simulink model "MMAE_beh_id_with_rel_LC_and_NGSIMTrajectories"  (R2018b)
settings: Solver=FixedStepAuto  StartTime=0.0  StopTime=90  FixedStep=Ts_bp  RelTol=1e-3
values from neighbouring files (symbols this model uses):
  ax = 0    [initialization.m]
  P_init = 1    [initialization.m]
  rel_x = 0    [initialization.m]
  Ts = 0.1    [KinematicBicycleModel.m]    (also in LeftLaneChangeSinusoidalMotionModel.m; LinearizedBicycleModel.m; SimplifiedKinematicBicycleModel.m; amm_rel_test.m)
  Ts_bp = 0.1    [initialization.m]    (also in laneChangeSinusoidalFcn.m = 0.01; laneChangeSinusoidalJacobianFcn.m = 0.01; leftLaneChangeParametricFcn.m = 0.01; leftLaneChangeParametricWithAccFcn.m = 0.01)
  vx = X(2)    [cv_model_fun.m]    (also in initialization.m = 10)
  vy = X(4)    [cv_model_fun.m]    (also in initialization.m = 0)
  x = X(1)    [KinematicBicycleModel.m]    (also in SimplifiedKinematicBicycleModel.m; behavior_model.m = 0:0.01:20; cca_model_fun.m; ctra_model_fun.m)
  y = X(2)    [KinematicBicycleModel.m]    (also in SimplifiedKinematicBicycleModel.m; behavior_model.m = [distances velocities]; cca_model_fun.m; ctra_model_fun.m)
undefined symbols (not defined in the file or in its folder): sigbuilder_block
libraries: simulink x8, dspswit3 x2, dspstat3 x2
settings Model: Creator=jasprit  LastModifiedBy=jasprit
settings SFSimCC: SimUseLocalCustomCode=off
settings RTWCC: RTWUseLocalCustomCode=off

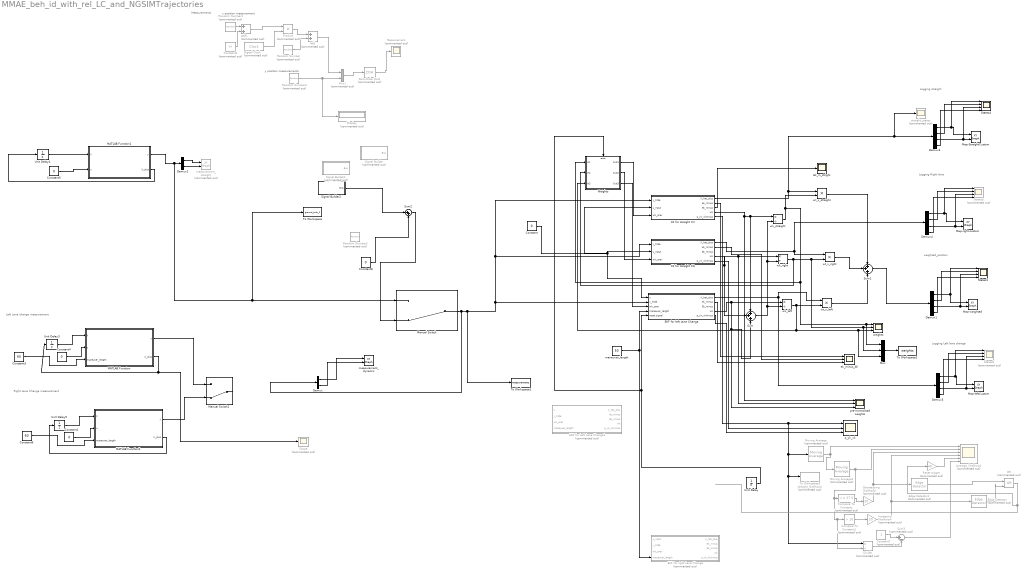
== system MMAE_beh_id_with_rel_LC_and_NGSIMTrajectories ==
  note: Left Lane change measurement
  note: Right Lane Change measurement
  note: Logging Left lane change
  note: Logging straight
  note: Logging Right lane
  note: y position measurements
  note: x position measurement
  note: Measurements
  note: weighted_position
  Add : Sum  Commented=on
  Add1 : Sum  Commented=on
  Average_likelihood : Scope  Commented=on  NumInputPorts=6
  Compare To Constant : simulink/Logic and Bit Operations/Compare To Constant  Commented=on  relop=<=  const=27.5  OutDataTypeStr=boolean
  Compare To Constant1 : simulink/Logic and Bit Operations/Compare To Constant  Commented=on  relop=>  const=10  OutDataTypeStr=boolean
  Constant : Constant  Value=0
  Constant1 : Constant  Value=0  SampleTime=-1
  Constant2 : Constant  Commented=on  Value=vx  SampleTime=Ts
  Constant3 : Constant  Value=60
  Constant4 : Constant  Value=0  SampleTime=-1
  Constant5 : Constant  Value=0  SampleTime=-1
  Constant6 : Constant  Value=60
  Constant7 : Constant  Commented=on
  Constant8 : Constant  Value=0
  Decreasomg likelihood : Gain  Commented=on  Gain=20
  Demux : Demux  Outputs=2
  Demux{1,3..5} (4 alike) : Demux
  Demux2 : Demux  Outputs=2
  Digital Clock : DigitalClock  Commented=on  SampleTime=Ts
  Display : Display  Commented=on
  Divide : Product  Commented=on  Inputs=*/
  EKF for Left Lane Change1 : Subsystem  Commented=on
  EKF for left Lane Change : Subsystem  TreatAsAtomicUnit=on
  EKF for right Lane Change : Subsystem  Commented=on
  Edge Detector : dspswit3/Edge Detector  Commented=on
      settings: SourceProductName=DSP System Toolbox  SourceProductBaseCode=DS
  Edge Detector1 : dspswit3/Edge Detector  Commented=on
      settings: SourceProductName=DSP System Toolbox  SourceProductBaseCode=DS
  Ek_m_stright : Scope
  Increasing likelihood : Gain  Commented=on  Gain=20
  KF for straight CA : Subsystem
  KF for straight CV : Subsystem
  MATLAB Function : MATLAB Function  TreatAsAtomicUnit=on
  MATLAB Function1 : MATLAB Function  TreatAsAtomicUnit=on
  MATLAB Function2 : MATLAB Function  TreatAsAtomicUnit=on
  Manual Switch : ManualSwitch  CurrentSetting=0
  Manual Switch1 : ManualSwitch  CurrentSetting=0
  Map-StraightCustom : simulink/Sinks/XY Graph  xmin=-1  xmax=200  ymin=-20  ymax=20  st=-1
  Map-leftCustom : simulink/Sinks/XY Graph  xmin=-1  xmax=300  ymin=-5  ymax=5  st=-1
  Map-right-custom : simulink/Sinks/XY Graph  xmin=-1  xmax=300  ymin=-5  ymax=5  st=-1
  Map-weighted : simulink/Sinks/XY Graph  xmin=-1  xmax=300  ymin=-5  ymax=5  st=-1
  "Measurement " : Scope  Commented=on
  Moving Average : dspstat3/Moving Average  Commented=on  Method=Sliding window  ForgettingFactorPort=off  SpecifyWindowLength=on  WindowLength=4  ForgettingFactor=0.9  SimulateUsing=Code generation
  Moving Average1 : dspstat3/Moving Average  Commented=on  Method=Sliding window  ForgettingFactorPort=off  SpecifyWindowLength=on  WindowLength=20  ForgettingFactor=0.9  SimulateUsing=Code generation
  Mux : Mux  Inputs=3
  Mux1 : Mux  Commented=on  Inputs=2
  OR : Logic  Commented=on  Operator=OR  IconShape=distinctive  AllPortsSameDT=off  OutDataTypeStr=boolean
  Product : Product  Commented=on
  Random Number : RandomNumber  Commented=on  Variance=0.0025  SampleTime=Ts
  Random Number1 : RandomNumber  Commented=on  Variance=0.0025  SampleTime=Ts
  Random Number2 : RandomNumber  Commented=on  Variance=0.0025  SampleTime=0.01
  Random Number3 : RandomNumber  Commented=on  Variance=0.0025  SampleTime=Ts
  Reset trigger : Gain  Commented=on  Gain=40
  Scope : Scope  Commented=on
  Signal Builder : Subsystem  Tag=STV Subsys  Commented=on  LoadFcn=sigbuilder_block('load');  StartFcn=sigbuilder_block('start');  StopFcn=sigbuilder_block('stop');  ClipboardFcn=sigbuilder_block('clipboard');  mask(Sigbuilder block){tuvar=[0:10]}
      mask help: Simulink:masks:SigbuilderBlock_MD
      mask init:
      | if ~strcmp(get_param(bdroot(gcbh),'SimulationStatus'),'stopped') tuvar = sigbuilder_block('maskInit'); end
      settings: CopyFcn=sigbuilder_block('copy');  DeleteFcn=sigbuilder_block('delete');  ModelCloseFcn=sigbuilder_block('modelClose');  PreSaveFcn=sigbuilder_block('preSave');  PauseFcn=sigbuilder_block('pause');  ContinueFcn=sigbuilder_block('continue');  NameChangeFcn=sigbuilder_block('namechange');  OpenFcn=sigbuilder_block('open',[414.75 96.75 558 422.25 ]);  CloseFcn=sigbuilder_block('close');
      mask Display: plot(0, 0, 100, 100,[2, 2, 32, 32, 2], [68, 8, 8, 68, 68],[32, 2], [38, 38], [32, 19, 2],[53, 60, 44], [32, 17, 17, 2],[16, 16, 31, 31]);txt = getActiveGroup(gcbh);text(2, 100, txt,'verticalAlignment', 'top');
  Signal Builder1 : Subsystem  Tag=STV Subsys  Commented=on  LoadFcn=sigbuilder_block('load');  StartFcn=sigbuilder_block('start');  StopFcn=sigbuilder_block('stop');  ClipboardFcn=sigbuilder_block('clipboard');  mask(Sigbuilder block){tuvar=[0:10]}
      mask help: Simulink:masks:SigbuilderBlock_MD
      mask init:
      | if ~strcmp(get_param(bdroot(gcbh),'SimulationStatus'),'stopped') tuvar = sigbuilder_block('maskInit'); end
      settings: CopyFcn=sigbuilder_block('copy');  DeleteFcn=sigbuilder_block('delete');  ModelCloseFcn=sigbuilder_block('modelClose');  PreSaveFcn=sigbuilder_block('preSave');  PauseFcn=sigbuilder_block('pause');  ContinueFcn=sigbuilder_block('continue');  NameChangeFcn=sigbuilder_block('namechange');  OpenFcn=sigbuilder_block('open',[492.75 131.25 580.5 283.5 ]);  CloseFcn=sigbuilder_block('close');
      mask Display: plot(0, 0, 100, 100,[2, 2, 32, 32, 2], [68, 8, 8, 68, 68],[32, 2], [38, 38], [32, 19, 2],[53, 60, 44], [32, 17, 17, 2],[16, 16, 31, 31]);txt = getActiveGroup(gcbh);text(2, 100, txt,'verticalAlignment', 'top');
  Signal Builder2 : Subsystem  Tag=STV Subsys  LoadFcn=sigbuilder_block('load');  StartFcn=sigbuilder_block('start');  StopFcn=sigbuilder_block('stop');  ClipboardFcn=sigbuilder_block('clipboard');  mask(Sigbuilder block){tuvar=[0:10]}
      mask help: Simulink:masks:SigbuilderBlock_MD
      mask init:
      | if ~strcmp(get_param(bdroot(gcbh),'SimulationStatus'),'stopped') tuvar = sigbuilder_block('maskInit'); end
      settings: CopyFcn=sigbuilder_block('copy');  DeleteFcn=sigbuilder_block('delete');  ModelCloseFcn=sigbuilder_block('modelClose');  PreSaveFcn=sigbuilder_block('preSave');  PauseFcn=sigbuilder_block('pause');  ContinueFcn=sigbuilder_block('continue');  NameChangeFcn=sigbuilder_block('namechange');  OpenFcn=sigbuilder_block('open',[437.6 178.5 550.15 399.75 ]);  CloseFcn=sigbuilder_block('close');
      mask Display: plot(0, 0, 100, 100,[2, 2, 32, 32, 2], [68, 8, 8, 68, 68],[32, 2], [38, 38], [32, 19, 2],[53, 60, 44], [32, 17, 17, 2],[16, 16, 31, 31]);txt = getActiveGroup(gcbh);text(2, 100, txt,'verticalAlignment', 'top');
  States1 : Scope  NumInputPorts=4
  States4 : Scope  NumInputPorts=4
  States5 : Scope  Commented=on  NumInputPorts=4
  States6 : Scope  Commented=on  NumInputPorts=4
  Sum : Sum  Inputs=+++
  Sum1 : Sum  Inputs=+++
  Sum2 : Sum  Inputs=|++
  Sum3 : Sum  Commented=on  Inputs=|+-
  To Workspace : ToWorkspace  VariableName=ground_truth_2  SaveFormat=Timeseries  SampleTime=-1
  To Workspace1 : ToWorkspace  VariableName=measurements  SaveFormat=Timeseries  SampleTime=-1
  To Workspace2 : ToWorkspace  VariableName=weights  SaveFormat=Timeseries  SampleTime=-1
  To Workspace3 : ToWorkspace  Commented=on  VariableName=straight_likelihood  SaveFormat=Timeseries  SampleTime=-1
  Unit Delay : UnitDelay  SampleTime=-1
  Unit Delay3 : UnitDelay  InitialCondition=[x vx y vy]  SampleTime=Ts_bp
  Unit Delay4 : UnitDelay  InitialCondition=[x vx y vy]  SampleTime=-1
  Unit Delay5 : UnitDelay  InitialCondition=[x vx y vy]  SampleTime=Ts_bp
  Weights : Subsystem
  Zero-Order Hold : ZeroOrderHold  Commented=on  SampleTime=Ts
  ek_minus_All : Scope  NumInputPorts=3
  maneuver_length : Constant  Value=50
  measurement_dynamic : simulink/Sinks/XY Graph  xmin=-1  xmax=700  ymin=-5  ymax=20  st=-1
  measurement_straight : simulink/Sinks/XY Graph  Commented=on  xmin=-1  xmax=200  ymin=-5  ymax=5  st=-1
  p_yk_xk : Scope  NumInputPorts=3
  pre-normalized weights : Scope  NumInputPorts=3
  straight_states : Scope  Commented=on
  weights : Scope  NumInputPorts=3
  wk_left : Product  Inputs=*/
  wk_right : Product  Inputs=*/
  wk_straight : Product  Inputs=*/
  wt_x_left : Product  Inputs=**
  wt_x_right : Product  Inputs=**
  wt_x_straight : Product  Inputs=**
  wires:
  Constant2/1 -> Add1/2
  Digital Clock/1 -> Product/2
  Product/1 -> Add/1
  Random Number/1 -> Add/2
  Add/1 -> Mux1/1
  Mux1/1 -> Zero-Order Hold/1
  Random Number3/1 -> Display/1, Mux1/2
  Zero-Order Hold/1 -> "Measurement "/1
  Demux3/1 -> States4/1, Map-StraightCustom/1
  Demux3/4 -> States4/4
  Demux3/2 -> States4/2
  Demux3/3 -> Map-StraightCustom/2, States4/3
  Constant/1 -> EKF for left Lane Change/1(u), KF for straight CA/2(u_input), KF for straight CV/2(u_input)
  Demux4/1 -> States5/1, Map-right-custom/1
  Demux4/2 -> States5/2
  Demux4/4 -> States5/4
  Demux4/3 -> Map-right-custom/2, States5/3
  Demux5/1 -> States6/1, Map-leftCustom/1
  Demux5/4 -> States6/4
  Demux5/3 -> Map-leftCustom/2, States6/3
  Demux5/2 -> States6/2
  EKF for left Lane Change/1(X_hat_plus) -> wt_x_left/1, Demux5/1
  KF for straight CA/1(X_hat_plus) -> Demux4/1, wt_x_right/1
  KF for straight CV/1(X_hat_plus) -> straight_states/1, Demux3/1, wt_x_straight/1
  EKF for left Lane Change/4(wk) -> wk_left/1, pre-normalized weights/3, Sum/3
  KF for straight CA/4(wk) -> pre-normalized weights/2, wk_right/1, Sum/2
  KF for straight CV/4(wk) -> pre-normalized weights/1, wk_straight/1, Sum/1
  Sum/1 -> wk_left/2, wk_straight/2, wk_right/2
  wk_straight/1 -> Weights/1(In1), Mux/1, weights/1, wt_x_straight/2
  wk_right/1 -> Weights/2(In2), Mux/2, weights/2, wt_x_right/2
  wk_left/1 -> Mux/3, weights/3, Weights/3(In3), wt_x_left/2
  wt_x_right/1 -> Sum1/2
  wt_x_straight/1 -> Sum1/1
  wt_x_left/1 -> Sum1/3
  Demux1/1 -> States1/1, Map-weighted/1
  Demux1/4 -> States1/4
  Demux1/2 -> States1/2
  Demux1/3 -> States1/3, Map-weighted/2
  Sum1/1 -> Demux1/1
  KF for straight CV/2(ek_minus) -> ek_minus_All/1
  KF for straight CA/2(ek_minus) -> ek_minus_All/2
  EKF for left Lane Change/2(ek_minus) -> ek_minus_All/3
  KF for straight CV/5(p_yk_xkminus) -> Moving Average/1, Divide/1, To Workspace3/1, p_yk_xk/1
  KF for straight CA/5(p_yk_xkminus) -> p_yk_xk/2
  EKF for left Lane Change/5(p_yk_xkminus) -> p_yk_xk/3
  KF for straight CV/3(Ek_minus) -> Ek_m_stright/1
  Manual Switch/1 -> To Workspace1/1, KF for straight CA/1(y_tilde), KF for straight CV/1(y_tilde), EKF for left Lane Change/2(y_tilde), Demux/1
  Unit Delay3/1 -> MATLAB Function/1(X)
  Constant4/1 -> MATLAB Function/2(u)
  Demux/1 -> measurement_dynamic/1
  Demux/2 -> measurement_dynamic/2
  MATLAB Function1/2(X_plus) -> Unit Delay4/1
  Constant5/1 -> MATLAB Function1/2(u)
  Unit Delay4/1 -> MATLAB Function1/1(X)
  MATLAB Function1/1(y) -> To Workspace/1, Manual Switch/1, Demux2/1
  Demux2/1 -> measurement_straight/1
  Demux2/2 -> measurement_straight/2
  MATLAB Function2/2(X_plus) -> Unit Delay5/1
  Unit Delay5/1 -> MATLAB Function2/1(X)
  Constant1/1 -> MATLAB Function2/2(u)
  MATLAB Function/1(y) -> Manual Switch1/1
  MATLAB Function2/1(y) -> Manual Switch1/2
  Random Number1/1 -> Add1/1
  Add1/1 -> Product/1
  maneuver_length/1 -> EKF for left Lane Change/4(maneuver_length), EKF for right Lane Change/4(maneuver_length)
  Constant3/1 -> MATLAB Function/3(maneuver_length)
  Constant6/1 -> MATLAB Function2/3(maneuver_length)
  MATLAB Function/2(X_plus) -> Scope/1, Unit Delay3/1
  Mux/1 -> To Workspace2/1
  Signal Builder2/1(Bus) -> Sum2/1
  Constant8/1 -> Sum2/2
  Sum2/1 -> Manual Switch/2
  Moving Average/1 -> Average_likelihood/1, Moving Average1/1
  Moving Average1/1 -> Divide/2, Compare To Constant1/1, Compare To Constant/1, Average_likelihood/2
  Decreasomg likelihood/1 -> Edge Detector1/1, Average_likelihood/3
  Unit Delay/1 -> Weights/Reset, EKF for left Lane Change/5(reset signal)
  Weights/1(Out1) -> KF for straight CV/3(wk_prev)
  Weights/2(Out2) -> KF for straight CA/3(wk_prev)
  Weights/3(Out3) -> EKF for left Lane Change/3(wk_prev)
  Compare To Constant/1 -> Decreasomg likelihood/1
  Compare To Constant1/1 -> Increasing likelihood/1
  Increasing likelihood/1 -> Edge Detector/1, Average_likelihood/4
  Edge Detector/1 -> OR/2
  Reset trigger/1 -> Average_likelihood/5
  Edge Detector1/1 -> OR/1
  OR/1 -> Reset trigger/1
  Constant7/1 -> Sum3/1
  Divide/1 -> Sum3/2
  Sum3/1 -> Average_likelihood/6

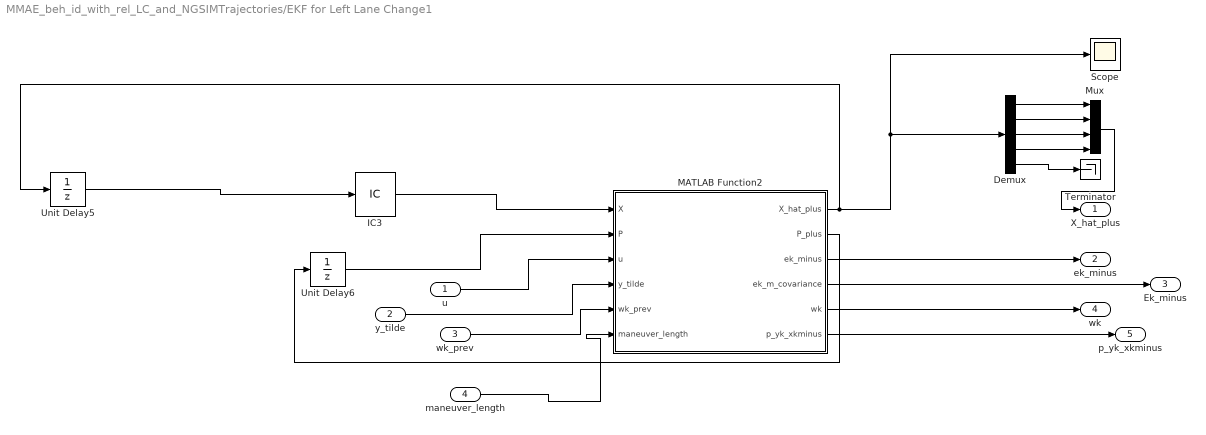
== system MMAE_beh_id_with_rel_LC_and_NGSIMTrajectories/EKF for Left Lane Change1 ==
  u : Inport
  y_tilde : Inport  Port=2
  wk_prev : Inport  Port=3
  maneuver_length : Inport  Port=4
  Demux : Demux  Outputs=5
  IC3 : InitialCondition  Value=[x vx y vy rel_x]
  MATLAB Function2 : MATLAB Function  TreatAsAtomicUnit=on
  Mux : Mux
  Scope : Scope
  Terminator : Terminator
  Unit Delay5 : UnitDelay  SampleTime=-1
  Unit Delay6 : UnitDelay  InitialCondition=diag([P_init, P_init, P_init, P_init, 200])  SampleTime=-1
  X_hat_plus : Outport
  ek_minus : Outport  Port=2
  Ek_minus : Outport  Port=3
  wk : Outport  Port=4
  p_yk_xkminus : Outport  Port=5
  wires:
  MATLAB Function2/2(P_plus) -> Unit Delay6/1
  u/1 -> MATLAB Function2/3(u)
  Unit Delay5/1 -> IC3/1
  y_tilde/1 -> MATLAB Function2/4(y_tilde)
  MATLAB Function2/1(X_hat_plus) -> Demux/1, Scope/1, Unit Delay5/1
  IC3/1 -> MATLAB Function2/1(X)
  Unit Delay6/1 -> MATLAB Function2/2(P)
  MATLAB Function2/3(ek_minus) -> ek_minus/1
  MATLAB Function2/4(ek_m_covariance) -> Ek_minus/1
  MATLAB Function2/5(wk) -> wk/1
  MATLAB Function2/6(p_yk_xkminus) -> p_yk_xkminus/1
  wk_prev/1 -> MATLAB Function2/5(wk_prev)
  maneuver_length/1 -> MATLAB Function2/6(maneuver_length)
  Demux/1 -> Mux/1
  Demux/2 -> Mux/2
  Demux/3 -> Mux/3
  Demux/4 -> Mux/4
  Demux/5 -> Terminator/1
  Mux/1 -> X_hat_plus/1

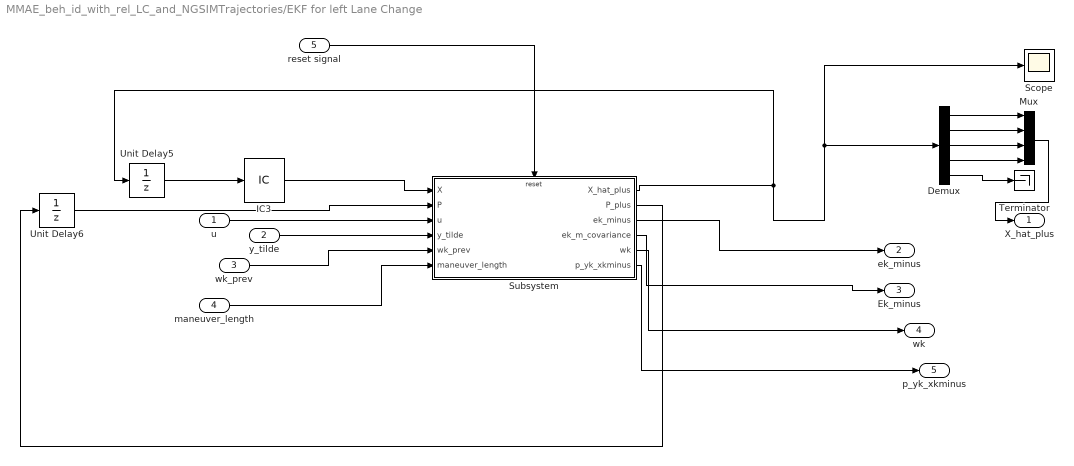
== system MMAE_beh_id_with_rel_LC_and_NGSIMTrajectories/EKF for left Lane Change ==
  u : Inport
  y_tilde : Inport  Port=2
  wk_prev : Inport  Port=3
  maneuver_length : Inport  Port=4
  reset signal : Inport  Port=5
  Demux : Demux  Outputs=5
  IC3 : InitialCondition  Value=[x vx y vy rel_x]
  Mux : Mux
  Scope : Scope
  Subsystem : Subsystem
  Terminator : Terminator
  Unit Delay5 : UnitDelay  InitialCondition=[x vx y vy rel_x]  SampleTime=-1
  Unit Delay6 : UnitDelay  InitialCondition=diag([P_init, P_init, P_init, P_init, 200])  SampleTime=-1
  X_hat_plus : Outport
  ek_minus : Outport  Port=2
  Ek_minus : Outport  Port=3
  wk : Outport  Port=4
  p_yk_xkminus : Outport  Port=5
  wires:
  Mux/1 -> X_hat_plus/1
  Demux/4 -> Mux/4
  Demux/5 -> Terminator/1
  Demux/3 -> Mux/3
  Demux/2 -> Mux/2
  Unit Delay5/1 -> IC3/1
  Demux/1 -> Mux/1
  Subsystem/1(X_hat_plus) -> Demux/1, Scope/1, Unit Delay5/1
  IC3/1 -> Subsystem/1(X)
  u/1 -> Subsystem/3(u)
  y_tilde/1 -> Subsystem/4(y_tilde)
  wk_prev/1 -> Subsystem/5(wk_prev)
  maneuver_length/1 -> Subsystem/6(maneuver_length)
  Subsystem/3(ek_minus) -> ek_minus/1
  Subsystem/4(ek_m_covariance) -> Ek_minus/1
  Subsystem/5(wk) -> wk/1
  Subsystem/6(p_yk_xkminus) -> p_yk_xkminus/1
  Unit Delay6/1 -> Subsystem/2(P)
  Subsystem/2(P_plus) -> Unit Delay6/1
  reset signal/1 -> Subsystem/Reset

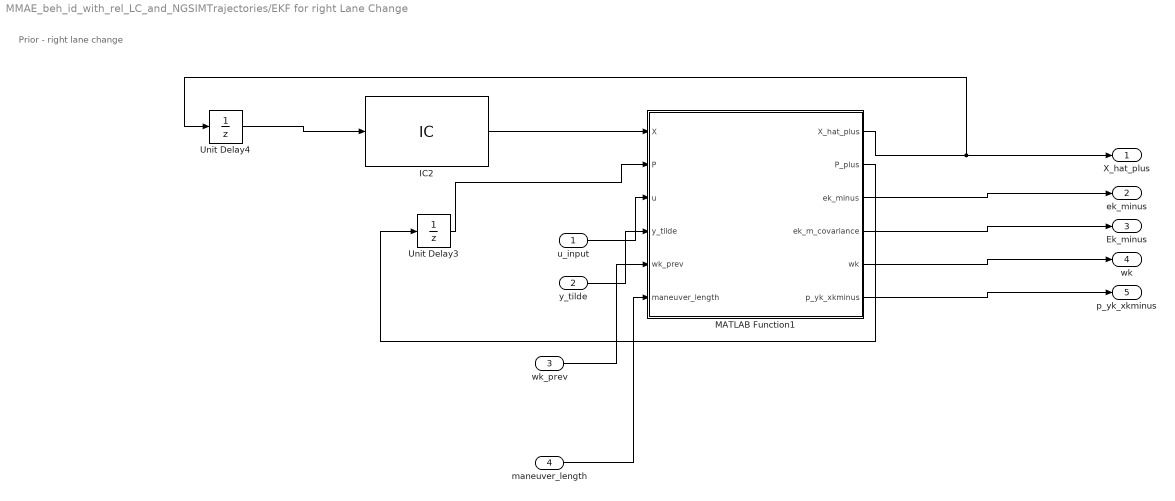
== system MMAE_beh_id_with_rel_LC_and_NGSIMTrajectories/EKF for right Lane Change ==
  note: Prior - right lane change
  u_input : Inport
  y_tilde : Inport  Port=2
  wk_prev : Inport  Port=3
  maneuver_length : Inport  Port=4
  IC2 : InitialCondition  Value=[x vx y vy]
  MATLAB Function1 : MATLAB Function  TreatAsAtomicUnit=on
  Unit Delay3 : UnitDelay  InitialCondition=eye(4)*P_init  SampleTime=-1
  Unit Delay4 : UnitDelay  SampleTime=-1
  X_hat_plus : Outport
  ek_minus : Outport  Port=2
  Ek_minus : Outport  Port=3
  wk : Outport  Port=4
  p_yk_xkminus : Outport  Port=5
  wires:
  MATLAB Function1/2(P_plus) -> Unit Delay3/1
  IC2/1 -> MATLAB Function1/1(X)
  Unit Delay3/1 -> MATLAB Function1/2(P)
  MATLAB Function1/1(X_hat_plus) -> X_hat_plus/1, Unit Delay4/1
  u_input/1 -> MATLAB Function1/3(u)
  y_tilde/1 -> MATLAB Function1/4(y_tilde)
  Unit Delay4/1 -> IC2/1
  MATLAB Function1/3(ek_minus) -> ek_minus/1
  MATLAB Function1/4(ek_m_covariance) -> Ek_minus/1
  wk_prev/1 -> MATLAB Function1/5(wk_prev)
  MATLAB Function1/5(wk) -> wk/1
  MATLAB Function1/6(p_yk_xkminus) -> p_yk_xkminus/1
  maneuver_length/1 -> MATLAB Function1/6(maneuver_length)

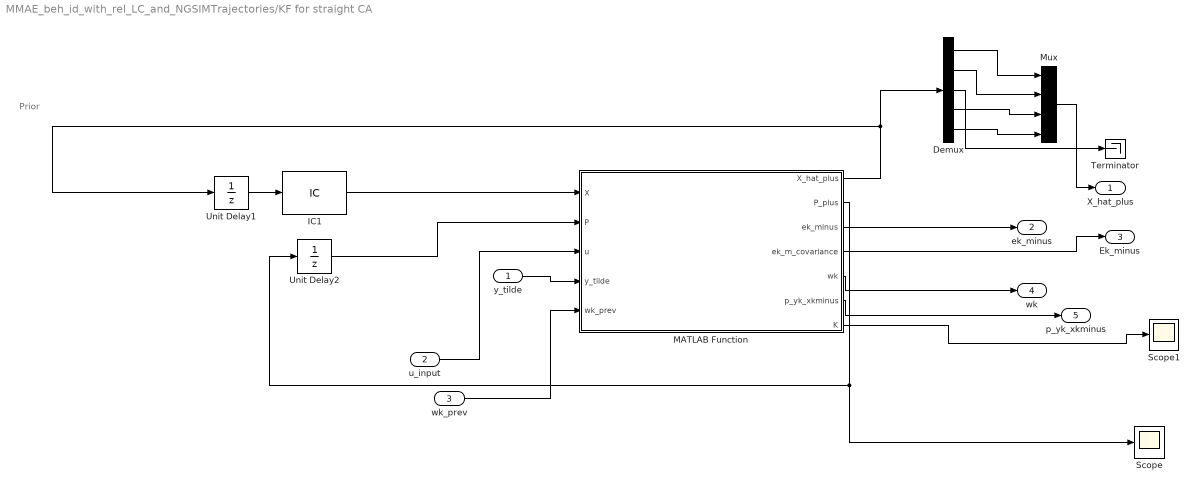
== system MMAE_beh_id_with_rel_LC_and_NGSIMTrajectories/KF for straight CA ==
  note: Prior
  y_tilde : Inport
  u_input : Inport  Port=2
  wk_prev : Inport  Port=3
  Demux : Demux  Outputs=5
  IC1 : InitialCondition  Value=[x vx ax y vy]
  MATLAB Function : MATLAB Function  TreatAsAtomicUnit=on
  Mux : Mux
  Scope : Scope
  Scope1 : Scope
  Terminator : Terminator
  Unit Delay1 : UnitDelay  SampleTime=-1
  Unit Delay2 : UnitDelay  InitialCondition=eye(5)*P_init  SampleTime=-1
  X_hat_plus : Outport
  ek_minus : Outport  Port=2
  Ek_minus : Outport  Port=3
  wk : Outport  Port=4
  p_yk_xkminus : Outport  Port=5
  wires:
  Unit Delay2/1 -> MATLAB Function/2(P)
  IC1/1 -> MATLAB Function/1(X)
  MATLAB Function/1(X_hat_plus) -> Demux/1, Unit Delay1/1
  u_input/1 -> MATLAB Function/3(u)
  Unit Delay1/1 -> IC1/1
  y_tilde/1 -> MATLAB Function/4(y_tilde)
  MATLAB Function/2(P_plus) -> Scope/1, Unit Delay2/1
  MATLAB Function/3(ek_minus) -> ek_minus/1
  MATLAB Function/4(ek_m_covariance) -> Ek_minus/1
  wk_prev/1 -> MATLAB Function/5(wk_prev)
  MATLAB Function/5(wk) -> wk/1
  MATLAB Function/6(p_yk_xkminus) -> p_yk_xkminus/1
  MATLAB Function/7(K) -> Scope1/1
  Demux/1 -> Mux/1
  Demux/2 -> Mux/2
  Demux/4 -> Mux/3
  Demux/5 -> Mux/4
  Demux/3 -> Terminator/1
  Mux/1 -> X_hat_plus/1

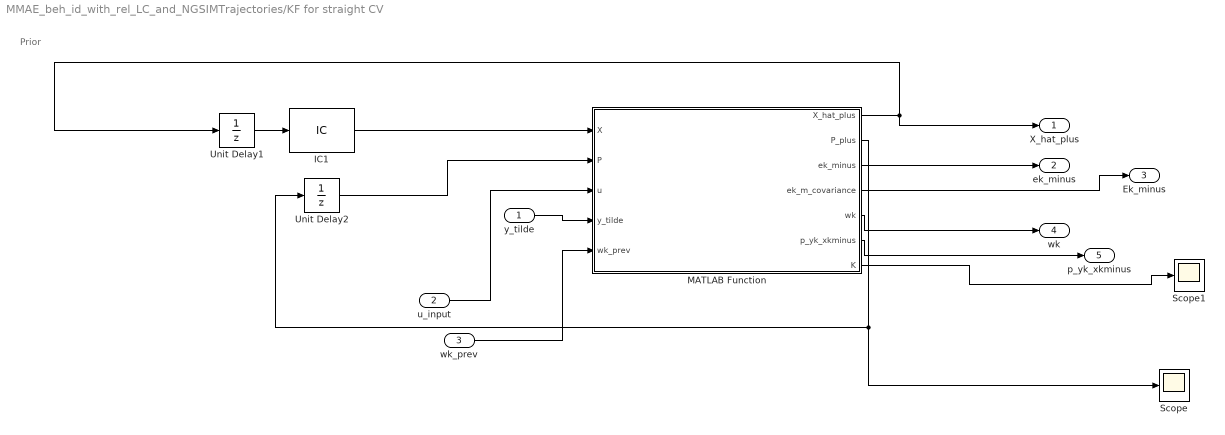
== system MMAE_beh_id_with_rel_LC_and_NGSIMTrajectories/KF for straight CV ==
  note: Prior
  y_tilde : Inport
  u_input : Inport  Port=2
  wk_prev : Inport  Port=3
  IC1 : InitialCondition  Value=[x vx y vy]
  MATLAB Function : MATLAB Function  TreatAsAtomicUnit=on
  Scope : Scope
  Scope1 : Scope
  Unit Delay1 : UnitDelay  SampleTime=-1
  Unit Delay2 : UnitDelay  InitialCondition=eye(4)*P_init  SampleTime=-1
  X_hat_plus : Outport
  ek_minus : Outport  Port=2
  Ek_minus : Outport  Port=3
  wk : Outport  Port=4
  p_yk_xkminus : Outport  Port=5
  wires:
  Unit Delay2/1 -> MATLAB Function/2(P)
  IC1/1 -> MATLAB Function/1(X)
  MATLAB Function/1(X_hat_plus) -> X_hat_plus/1, Unit Delay1/1
  u_input/1 -> MATLAB Function/3(u)
  Unit Delay1/1 -> IC1/1
  y_tilde/1 -> MATLAB Function/4(y_tilde)
  MATLAB Function/2(P_plus) -> Scope/1, Unit Delay2/1
  MATLAB Function/3(ek_minus) -> ek_minus/1
  MATLAB Function/4(ek_m_covariance) -> Ek_minus/1
  wk_prev/1 -> MATLAB Function/5(wk_prev)
  MATLAB Function/5(wk) -> wk/1
  MATLAB Function/6(p_yk_xkminus) -> p_yk_xkminus/1
  MATLAB Function/7(K) -> Scope1/1

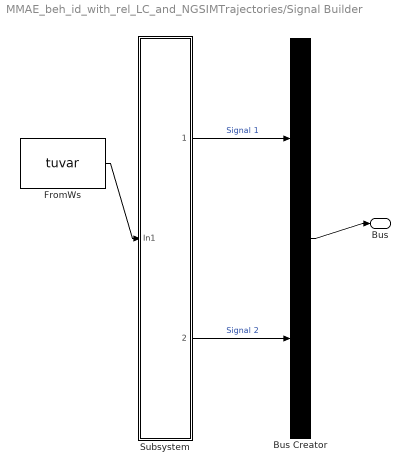
== system MMAE_beh_id_with_rel_LC_and_NGSIMTrajectories/Signal Builder ==
  Bus Creator : BusCreator  Tag=Bus Creator  Inputs=2
  FromWs : FromWorkspace  Tag=STV FromWs  VariableName=tuvar  SampleTime=0
  Subsystem : Subsystem
  Bus : Outport
  wires:
  FromWs/1 -> Subsystem/1(In1)
  Bus Creator/1 -> Bus/1
  Subsystem/1(Signal 1) -> Bus Creator/1  "Signal 1"
  Subsystem/2(Signal 2) -> Bus Creator/2  "Signal 2"

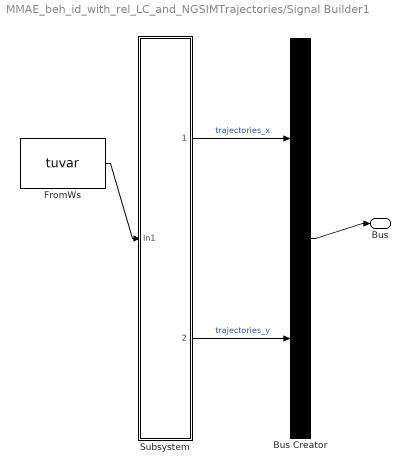
== system MMAE_beh_id_with_rel_LC_and_NGSIMTrajectories/Signal Builder1 ==
  Bus Creator : BusCreator  Tag=Bus Creator  Inputs=2
  FromWs : FromWorkspace  Tag=STV FromWs  VariableName=tuvar  SampleTime=0
  Subsystem : Subsystem
  Bus : Outport
  wires:
  FromWs/1 -> Subsystem/1(In1)
  Subsystem/1(trajectories_x) -> Bus Creator/1  "trajectories_x"
  Subsystem/2(trajectories_y) -> Bus Creator/2  "trajectories_y"
  Bus Creator/1 -> Bus/1

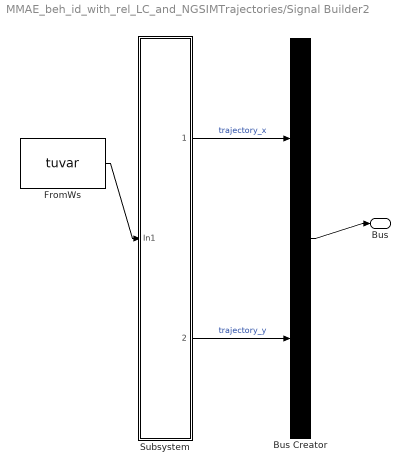
== system MMAE_beh_id_with_rel_LC_and_NGSIMTrajectories/Signal Builder2 ==
  Bus Creator : BusCreator  Tag=Bus Creator  Inputs=2
  FromWs : FromWorkspace  Tag=STV FromWs  VariableName=tuvar  SampleTime=0
      SigBuilderData=|
      | common.afterFinalStr = 'Extrapolate'
      | common.sampleTime = 0
      | dataSet.timeRange = [0 90]
      | dataSet.name = 'Group 1'
      | sbobj.Groups.Name = 'Group 1'
      | sbobj.Groups.Signals(1).Name = 'trajectory_x'
      | sbobj.Groups.Signals(1).XData = [0 0.1 0.2 0.3 0.4 0.5 0.6 0.7 0.8 0.9 1 1.1 ... (885 elements, 1x885)]
      | sbobj.Groups.Signals(1).YData = [14.6953224 15.0763224 15.4570176 15.8383224 16.2193224 16.6003224 16.9810176 17.3601888 17.7390552 18.1243224 18.5245248 18.9454536 ... (885 elements, 1x885)]
      | sbobj.Groups.Signals(2).Name = 'trajectory_y'
      | sbobj.Groups.Signals(2).XData = [0 0.1 0.2 0.3 0.4 0.5 0.6 0.7 0.8 0.9 1 1.1 ... (885 elements, 1x885)]
      | sbobj.Groups.Signals(2).YData = [23.40102 23.3845608 23.3684064 23.3519472 23.3357928 23.3196384 23.303484 23.2873296 23.2650792 23.277576 23.3056176 23.3574336 ... (885 elements, 1x885)]
      | sbobj.Groups.TimeRange = [0 90]
  Subsystem : Subsystem
  Bus : Outport
  wires:
  FromWs/1 -> Subsystem/1(In1)
  Bus Creator/1 -> Bus/1
  Subsystem/1(trajectory_x) -> Bus Creator/1  "trajectory_x"
  Subsystem/2(trajectory_y) -> Bus Creator/2  "trajectory_y"

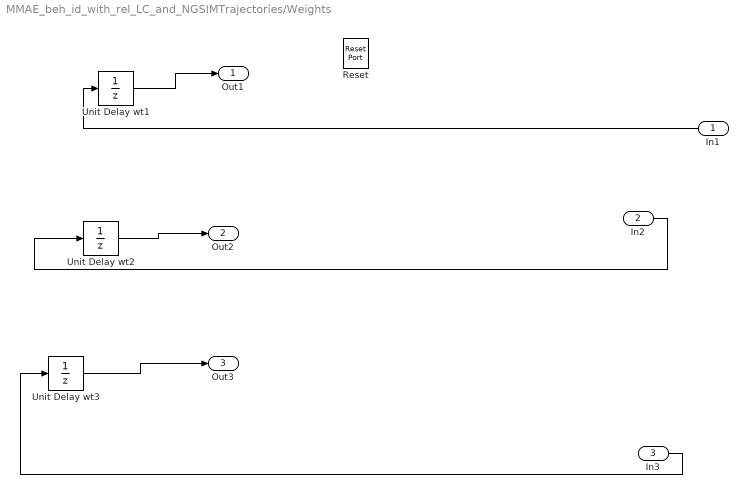
== system MMAE_beh_id_with_rel_LC_and_NGSIMTrajectories/Weights ==
  In1 : Inport
  In2 : Inport  Port=2
  In3 : Inport  Port=3
  Reset : ResetPort  DisableCoverage=on
  Unit Delay wt1 : UnitDelay  InitialCondition=1/3  SampleTime=-1
  Unit Delay wt2 : UnitDelay  InitialCondition=1/3  SampleTime=-1
  Unit Delay wt3 : UnitDelay  InitialCondition=1/3  SampleTime=-1
  Out1 : Outport
  Out2 : Outport  Port=2
  Out3 : Outport  Port=3
  wires:
  In1/1 -> Unit Delay wt1/1
  Unit Delay wt1/1 -> Out1/1
  In2/1 -> Unit Delay wt2/1
  Unit Delay wt2/1 -> Out2/1
  Unit Delay wt3/1 -> Out3/1
  In3/1 -> Unit Delay wt3/1

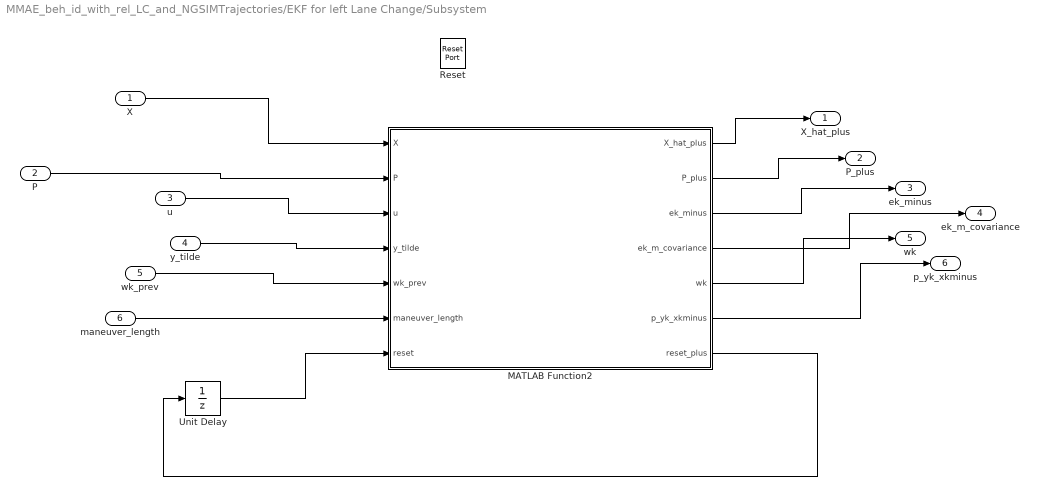
== system MMAE_beh_id_with_rel_LC_and_NGSIMTrajectories/EKF for left Lane Change/Subsystem ==
  X : Inport
  P : Inport  Port=2
  u : Inport  Port=3
  y_tilde : Inport  Port=4
  wk_prev : Inport  Port=5
  maneuver_length : Inport  Port=6
  Reset : ResetPort  DisableCoverage=on
  MATLAB Function2 : MATLAB Function  TreatAsAtomicUnit=on
  Unit Delay : UnitDelay  InitialCondition=1  SampleTime=-1
  X_hat_plus : Outport
  P_plus : Outport  Port=2
  ek_minus : Outport  Port=3
  ek_m_covariance : Outport  Port=4
  wk : Outport  Port=5
  p_yk_xkminus : Outport  Port=6
  wires:
  MATLAB Function2/5(wk) -> wk/1
  MATLAB Function2/1(X_hat_plus) -> X_hat_plus/1
  X/1 -> MATLAB Function2/1(X)
  P/1 -> MATLAB Function2/2(P)
  u/1 -> MATLAB Function2/3(u)
  wk_prev/1 -> MATLAB Function2/5(wk_prev)
  MATLAB Function2/3(ek_minus) -> ek_minus/1
  y_tilde/1 -> MATLAB Function2/4(y_tilde)
  maneuver_length/1 -> MATLAB Function2/6(maneuver_length)
  MATLAB Function2/2(P_plus) -> P_plus/1
  MATLAB Function2/6(p_yk_xkminus) -> p_yk_xkminus/1
  MATLAB Function2/4(ek_m_covariance) -> ek_m_covariance/1
  Unit Delay/1 -> MATLAB Function2/7(reset)
  MATLAB Function2/7(reset_plus) -> Unit Delay/1

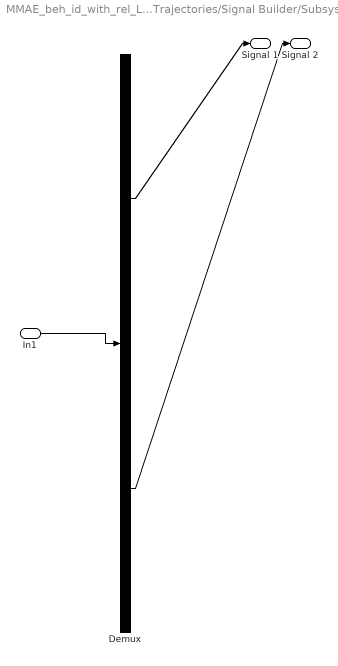
== system MMAE_beh_id_with_rel_LC_and_NGSIMTrajectories/Signal Builder/Subsystem ==
  In1 : Inport
  Demux : Demux  Tag=STV Demux  Outputs=2
  Signal 1 : Outport  Tag=STV Outport
  Signal 2 : Outport  Tag=STV Outport  Port=2
  wires:
  In1/1 -> Demux/1
  Demux/1 -> Signal 1/1
  Demux/2 -> Signal 2/1

== system MMAE_beh_id_with_rel_LC_and_NGSIMTrajectories/Signal Builder1/Subsystem ==
  In1 : Inport
  Demux : Demux  Tag=STV Demux  Outputs=2
  trajectories_x : Outport  Tag=STV Outport
  trajectories_y : Outport  Tag=STV Outport  Port=2
  wires:
  Demux/1 -> trajectories_x/1
  Demux/2 -> trajectories_y/1
  In1/1 -> Demux/1

== system MMAE_beh_id_with_rel_LC_and_NGSIMTrajectories/Signal Builder2/Subsystem ==
  In1 : Inport
  Demux : Demux  Tag=STV Demux  Outputs=2
  trajectory_x : Outport  Tag=STV Outport
  trajectory_y : Outport  Tag=STV Outport  Port=2
  wires:
  In1/1 -> Demux/1
  Demux/1 -> trajectory_x/1
  Demux/2 -> trajectory_y/1
